simulink library "DatalogHandler"  (R2016b)
settings: Solver=VariableStepAuto  StartTime=0.0  StopTime=10.0  RelTol=1e-3
libraries: VariousLibrary x6, ConversionsLibrary x6, slrtlib x1
(part 1 of 2)
settings Model: Creator=march  LastModifiedBy=march

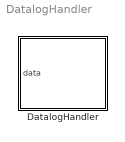
== system DatalogHandler ==
  DatalogHandler : Subsystem

== system DatalogHandler/DatalogHandler ==
  data : Inport
  Bus Selector1 : BusSelector  OutputSignals=etherCATData.receivedFromSOMANETs,etherCATData.sendToSOMANETs,miscDataSOMANETs.jointControlConfigs,miscDataSOMANETs.somanetData,etherCATData.receivedFromGESs,etherCATData.receivedFromInputDevice,etherCATData.sendToInputDevice,etherCATData.receivedFromPowerElectronics,etherCATData.sendToPowerElectronics,error,masterState,errorMessage
  "DataLogger " : slrtlib/Displays and Logging/Scope   scopeno=10  scopetype=File  autostart=on  viewmode=Graphical redraw  formatstr='%15.6f'  grid=on  ylimits=[0,0]  nosamples=900000  noprepostsamples=0  interleave=1  triggermode=FreeRun  triggersignal=1  trigsignalfromport=off  triggerlevel=0.0  triggerslope=Either  triggerscope=1  triggersample=0  filename=MARCH<%%>.dat  mode=Lazy  writesize=512  autorestart=on  dynamicfilemode=on  maxwritefilesize=512*1024^2
  Mux : Mux  Inputs=193
  Subsystem : Subsystem
  wires:
  Mux/1 -> "DataLogger "/1
  Subsystem/193(Out193) -> Mux/193
  Subsystem/192(Out192) -> Mux/192
  Subsystem/191(Out191) -> Mux/191
  Subsystem/190(Out190) -> Mux/190
  Subsystem/189(Out189) -> Mux/189
  Subsystem/188(Out188) -> Mux/188
  Subsystem/187(Out187) -> Mux/187
  Subsystem/186(Out186) -> Mux/186
  Subsystem/185(Out185) -> Mux/185
  Subsystem/184(Out184) -> Mux/184
  Subsystem/183(Out183) -> Mux/183
  Subsystem/182(Out182) -> Mux/182
  Subsystem/181(Out181) -> Mux/181
  Subsystem/180(Out180) -> Mux/180
  Subsystem/179(Out179) -> Mux/179
  Subsystem/178(Out178) -> Mux/178
  Subsystem/177(Out177) -> Mux/177
  Subsystem/176(Out176) -> Mux/176
  Subsystem/175(Out175) -> Mux/175
  Subsystem/174(Out174) -> Mux/174
  Subsystem/173(Out173) -> Mux/173
  Subsystem/172(Out172) -> Mux/172
  Subsystem/171(Out171) -> Mux/171
  Subsystem/170(Out170) -> Mux/170
  Subsystem/169(Out169) -> Mux/169
  Subsystem/168(Out168) -> Mux/168
  Subsystem/167(Out167) -> Mux/167
  Subsystem/166(Out166) -> Mux/166
  Subsystem/165(Out165) -> Mux/165
  Subsystem/164(Out164) -> Mux/164
  Subsystem/163(Out163) -> Mux/163
  Subsystem/162(Out162) -> Mux/162
  Subsystem/161(Out161) -> Mux/161
  Subsystem/160(Out160) -> Mux/160
  Subsystem/159(Out159) -> Mux/159
  Subsystem/158(Out158) -> Mux/158
  Subsystem/157(Out157) -> Mux/157
  Subsystem/156(Out156) -> Mux/156
  Subsystem/155(Out155) -> Mux/155
  Subsystem/154(Out154) -> Mux/154
  Subsystem/153(Out153) -> Mux/153
  Subsystem/152(Out152) -> Mux/152
  Subsystem/151(Out151) -> Mux/151
  Subsystem/150(Out150) -> Mux/150
  Subsystem/149(Out149) -> Mux/149
  Subsystem/148(Out148) -> Mux/148
  Subsystem/147(Out147) -> Mux/147
  Subsystem/146(Out146) -> Mux/146
  Subsystem/145(Out145) -> Mux/145
  Subsystem/144(Out144) -> Mux/144
  Subsystem/143(Out143) -> Mux/143
  Subsystem/142(Out142) -> Mux/142
  Subsystem/141(Out141) -> Mux/141
  Subsystem/140(Out140) -> Mux/140
  Subsystem/139(Out139) -> Mux/139
  Subsystem/138(Out138) -> Mux/138
  Subsystem/137(Out137) -> Mux/137
  Subsystem/136(Out136) -> Mux/136
  Subsystem/135(Out135) -> Mux/135
  Subsystem/134(Out134) -> Mux/134
  Subsystem/133(Out133) -> Mux/133
  Subsystem/132(Out132) -> Mux/132
  Subsystem/131(Out131) -> Mux/131
  Subsystem/130(Out130) -> Mux/130
  Subsystem/129(Out129) -> Mux/129
  Subsystem/128(Out128) -> Mux/128
  Subsystem/127(Out127) -> Mux/127
  Subsystem/126(Out126) -> Mux/126
  Subsystem/125(Out125) -> Mux/125
  Subsystem/124(Out124) -> Mux/124
  Subsystem/123(Out123) -> Mux/123
  Subsystem/122(Out122) -> Mux/122
  Subsystem/121(Out121) -> Mux/121
  Subsystem/120(Out120) -> Mux/120
  Subsystem/119(Out119) -> Mux/119
  Subsystem/118(Out118) -> Mux/118
  Subsystem/117(Out117) -> Mux/117
  Subsystem/116(Out116) -> Mux/116
  Subsystem/115(Out115) -> Mux/115
  Subsystem/114(Out114) -> Mux/114
  Subsystem/113(Out113) -> Mux/113
  Subsystem/112(Out112) -> Mux/112
  Subsystem/111(Out111) -> Mux/111
  Subsystem/110(Out110) -> Mux/110
  Subsystem/109(Out109) -> Mux/109
  Subsystem/108(Out108) -> Mux/108
  Subsystem/107(Out107) -> Mux/107
  Subsystem/106(Out106) -> Mux/106
  Subsystem/105(Out105) -> Mux/105
  Subsystem/104(Out104) -> Mux/104
  Subsystem/103(Out103) -> Mux/103
  Subsystem/102(Out102) -> Mux/102
  Subsystem/101(Out101) -> Mux/101
  Subsystem/100(Out100) -> Mux/100
  Subsystem/99(Out99) -> Mux/99
  Subsystem/98(Out98) -> Mux/98
  Subsystem/97(Out97) -> Mux/97
  Subsystem/96(Out96) -> Mux/96
  Subsystem/95(Out95) -> Mux/95
  Subsystem/94(Out94) -> Mux/94
  Subsystem/93(Out93) -> Mux/93
  Subsystem/92(Out92) -> Mux/92
  Subsystem/91(Out91) -> Mux/91
  Subsystem/90(Out90) -> Mux/90
  Subsystem/89(Out89) -> Mux/89
  Subsystem/88(Out88) -> Mux/88
  Subsystem/87(Out87) -> Mux/87
  Subsystem/86(Out86) -> Mux/86
  Subsystem/85(Out85) -> Mux/85
  Subsystem/84(Out84) -> Mux/84
  Subsystem/83(Out83) -> Mux/83
  Subsystem/82(Out82) -> Mux/82
  Subsystem/81(Out81) -> Mux/81
  Subsystem/80(Out80) -> Mux/80
  Subsystem/79(Out79) -> Mux/79
  Subsystem/78(Out78) -> Mux/78
  Subsystem/77(Out77) -> Mux/77
  Subsystem/76(Out76) -> Mux/76
  Subsystem/75(Out75) -> Mux/75
  Subsystem/74(Out74) -> Mux/74
  Subsystem/73(Out73) -> Mux/73
  Subsystem/72(Out72) -> Mux/72
  Subsystem/71(Out71) -> Mux/71
  Subsystem/70(Out70) -> Mux/70
  Subsystem/69(Out69) -> Mux/69
  Subsystem/68(Out68) -> Mux/68
  Subsystem/67(Out67) -> Mux/67
  Subsystem/66(Out66) -> Mux/66
  Subsystem/65(Out65) -> Mux/65
  Subsystem/64(Out64) -> Mux/64
  Subsystem/63(Out63) -> Mux/63
  Subsystem/62(Out62) -> Mux/62
  Subsystem/61(Out61) -> Mux/61
  Subsystem/60(Out60) -> Mux/60
  Subsystem/59(Out59) -> Mux/59
  Subsystem/58(Out58) -> Mux/58
  Subsystem/57(Out57) -> Mux/57
  Subsystem/56(Out56) -> Mux/56
  Subsystem/55(Out55) -> Mux/55
  Subsystem/54(Out54) -> Mux/54
  Subsystem/53(Out53) -> Mux/53
  Subsystem/52(Out52) -> Mux/52
  Subsystem/51(Out51) -> Mux/51
  Subsystem/50(Out50) -> Mux/50
  Subsystem/49(Out49) -> Mux/49
  Subsystem/48(Out48) -> Mux/48
  Subsystem/47(Out47) -> Mux/47
  Subsystem/46(Out46) -> Mux/46
  Subsystem/45(Out45) -> Mux/45
  Subsystem/44(Out44) -> Mux/44
  Subsystem/43(Out43) -> Mux/43
  Subsystem/42(Out42) -> Mux/42
  Subsystem/41(Out41) -> Mux/41
  Subsystem/40(Out40) -> Mux/40
  Subsystem/39(Out39) -> Mux/39
  Subsystem/38(Out38) -> Mux/38
  Subsystem/37(Out37) -> Mux/37
  Subsystem/36(Out36) -> Mux/36
  Subsystem/35(Out35) -> Mux/35
  Subsystem/34(Out34) -> Mux/34
  Subsystem/33(Out33) -> Mux/33
  Subsystem/32(Out32) -> Mux/32
  Subsystem/31(Out31) -> Mux/31
  Subsystem/30(Out30) -> Mux/30
  Subsystem/29(Out29) -> Mux/29
  Subsystem/28(Out28) -> Mux/28
  Subsystem/27(Out27) -> Mux/27
  Subsystem/26(Out26) -> Mux/26
  Subsystem/25(Out25) -> Mux/25
  Subsystem/24(Out24) -> Mux/24
  Subsystem/23(Out23) -> Mux/23
  Subsystem/22(Out22) -> Mux/22
  Subsystem/21(Out21) -> Mux/21
  Subsystem/20(Out20) -> Mux/20
  Subsystem/19(Out19) -> Mux/19
  Subsystem/18(Out18) -> Mux/18
  Subsystem/17(Out17) -> Mux/17
  Subsystem/16(Out16) -> Mux/16
  Subsystem/15(Out15) -> Mux/15
  Subsystem/14(Out14) -> Mux/14
  Subsystem/13(Out13) -> Mux/13
  Subsystem/12(Out12) -> Mux/12
  Subsystem/11(Out11) -> Mux/11
  Subsystem/10(Out10) -> Mux/10
  Subsystem/9(Out9) -> Mux/9
  Subsystem/8(Out8) -> Mux/8
  Subsystem/7(Out7) -> Mux/7
  Subsystem/6(Out6) -> Mux/6
  Subsystem/5(Out5) -> Mux/5
  Subsystem/4(Out4) -> Mux/4
  Subsystem/3(Out3) -> Mux/3
  Subsystem/2(Out2) -> Mux/2
  Subsystem/1(Out1) -> Mux/1
  Bus Selector1/12 -> Subsystem/12(In12)  "<errorMessage>"
  Bus Selector1/11 -> Subsystem/11(In11)  "<masterState>"
  Bus Selector1/10 -> Subsystem/10(In10)  "<error>"
  Bus Selector1/9 -> Subsystem/9(In9)  "<sendToPowerElectronics>"
  Bus Selector1/8 -> Subsystem/8(In8)  "<receivedFromPowerElectronics>"
  Bus Selector1/7 -> Subsystem/7(In7)  "<sendToInputDevice>"
  Bus Selector1/6 -> Subsystem/6(In6)  "<receivedFromInputDevice>"
  Bus Selector1/5 -> Subsystem/5(In5)  "<receivedFromGESs>"
  Bus Selector1/4 -> Subsystem/4(In4)  "<somanetData>"
  Bus Selector1/3 -> Subsystem/3(In3)  "<jointControlConfigs>"
  Bus Selector1/2 -> Subsystem/2(In2)  "<sendToSOMANETs>"
  Bus Selector1/1 -> Subsystem/1(In1)  "<receivedFromSOMANETs>"
  data/1 -> Bus Selector1/1

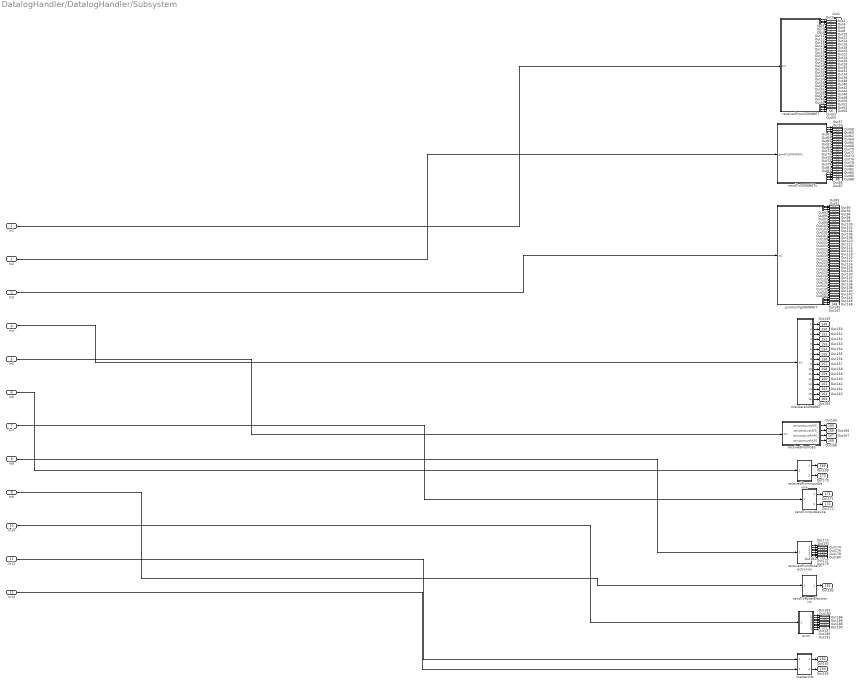
== system DatalogHandler/DatalogHandler/Subsystem ==
  In1 : Inport
  In2 : Inport  Port=2
  In3 : Inport  Port=3
  In4 : Inport  Port=4
  In5 : Inport  Port=5
  In6 : Inport  Port=6
  In7 : Inport  Port=7
  In8 : Inport  Port=8
  In9 : Inport  Port=9
  In10 : Inport  Port=10
  In11 : Inport  Port=11
  In12 : Inport  Port=12
  error : Subsystem
  jointConfigSOMANET : Subsystem
  masterInfo : Subsystem
  miscDataSOMANET : Subsystem
  receivedFromGES : Subsystem
  receivedFromInputDevice : Subsystem
  receivedFromPowerElectronics : Subsystem
  receivedFromSOMANET : Subsystem
  sendToInputDevice : Subsystem
  sendToPowerElectronics : Subsystem
  sendToSOMANETs : Subsystem
  Out1 : Outport
  Out2 : Outport  Port=2
  Out3 : Outport  Port=3
  Out4 : Outport  Port=4
  Out5 : Outport  Port=5
  Out6 : Outport  Port=6
  Out7 : Outport  Port=7
  Out8 : Outport  Port=8
  Out9 : Outport  Port=9
  Out10 : Outport  Port=10
  Out11 : Outport  Port=11
  Out12 : Outport  Port=12
  Out13 : Outport  Port=13
  Out14 : Outport  Port=14
  Out15 : Outport  Port=15
  Out16 : Outport  Port=16
  Out17 : Outport  Port=17
  Out18 : Outport  Port=18
  Out19 : Outport  Port=19
  Out20 : Outport  Port=20
  Out21 : Outport  Port=21
  Out22 : Outport  Port=22
  Out23 : Outport  Port=23
  Out24 : Outport  Port=24
  Out25 : Outport  Port=25
  Out26 : Outport  Port=26
  Out27 : Outport  Port=27
  Out28 : Outport  Port=28
  Out29 : Outport  Port=29
  Out30 : Outport  Port=30
  Out31 : Outport  Port=31
  Out32 : Outport  Port=32
  Out33 : Outport  Port=33
  Out34 : Outport  Port=34
  Out35 : Outport  Port=35
  Out36 : Outport  Port=36
  Out37 : Outport  Port=37
  Out38 : Outport  Port=38
  Out39 : Outport  Port=39
  Out40 : Outport  Port=40
  Out41 : Outport  Port=41
  Out42 : Outport  Port=42
  Out43 : Outport  Port=43
  Out44 : Outport  Port=44
  Out45 : Outport  Port=45
  Out46 : Outport  Port=46
  Out47 : Outport  Port=47
  Out48 : Outport  Port=48
  Out49 : Outport  Port=49
  Out50 : Outport  Port=50
  Out51 : Outport  Port=51
  Out52 : Outport  Port=52
  Out53 : Outport  Port=53
  Out54 : Outport  Port=54
  Out55 : Outport  Port=55
  Out56 : Outport  Port=56
  Out57 : Outport  Port=57
  Out58 : Outport  Port=58
  Out59 : Outport  Port=59
  Out60 : Outport  Port=60
  Out61 : Outport  Port=61
  Out62 : Outport  Port=62
  Out63 : Outport  Port=63
  Out64 : Outport  Port=64
  Out65 : Outport  Port=65
  Out66 : Outport  Port=66
  Out67 : Outport  Port=67
  Out68 : Outport  Port=68
  Out69 : Outport  Port=69
  Out70 : Outport  Port=70
  Out71 : Outport  Port=71
  Out72 : Outport  Port=72
  Out73 : Outport  Port=73
  Out74 : Outport  Port=74
  Out75 : Outport  Port=75
  Out76 : Outport  Port=76
  Out77 : Outport  Port=77
  Out78 : Outport  Port=78
  Out79 : Outport  Port=79
  Out80 : Outport  Port=80
  Out81 : Outport  Port=81
  Out82 : Outport  Port=82
  Out83 : Outport  Port=83
  Out84 : Outport  Port=84
  Out85 : Outport  Port=85
  Out86 : Outport  Port=86
  Out87 : Outport  Port=87
  Out88 : Outport  Port=88
  Out89 : Outport  Port=89
  Out90 : Outport  Port=90
  Out91 : Outport  Port=91
  Out92 : Outport  Port=92
  Out93 : Outport  Port=93
  Out94 : Outport  Port=94
  Out95 : Outport  Port=95
  Out96 : Outport  Port=96
  Out97 : Outport  Port=97
  Out98 : Outport  Port=98
  Out99 : Outport  Port=99
  Out100 : Outport  Port=100
  Out101 : Outport  Port=101
  Out102 : Outport  Port=102
  Out103 : Outport  Port=103
  Out104 : Outport  Port=104
  Out105 : Outport  Port=105
  Out106 : Outport  Port=106
  Out107 : Outport  Port=107
  Out108 : Outport  Port=108
  Out109 : Outport  Port=109
  Out110 : Outport  Port=110
  Out111 : Outport  Port=111
  Out112 : Outport  Port=112
  Out113 : Outport  Port=113
  Out114 : Outport  Port=114
  Out115 : Outport  Port=115
  Out116 : Outport  Port=116
  Out117 : Outport  Port=117
  Out118 : Outport  Port=118
  Out119 : Outport  Port=119
  Out120 : Outport  Port=120
  Out121 : Outport  Port=121
  Out122 : Outport  Port=122
  Out123 : Outport  Port=123
  Out124 : Outport  Port=124
  Out125 : Outport  Port=125
  Out126 : Outport  Port=126
  Out127 : Outport  Port=127
  Out128 : Outport  Port=128
  Out129 : Outport  Port=129
  Out130 : Outport  Port=130
  Out131 : Outport  Port=131
  Out132 : Outport  Port=132
  Out133 : Outport  Port=133
  Out134 : Outport  Port=134
  Out135 : Outport  Port=135
  Out136 : Outport  Port=136
  Out137 : Outport  Port=137
  Out138 : Outport  Port=138
  Out139 : Outport  Port=139
  Out140 : Outport  Port=140
  Out141 : Outport  Port=141
  Out142 : Outport  Port=142
  Out143 : Outport  Port=143
  Out144 : Outport  Port=144
  Out145 : Outport  Port=145
  Out146 : Outport  Port=146
  Out147 : Outport  Port=147
  Out148 : Outport  Port=148
  Out149 : Outport  Port=149
  Out150 : Outport  Port=150
  Out151 : Outport  Port=151
  Out152 : Outport  Port=152
  Out153 : Outport  Port=153
  Out154 : Outport  Port=154
  Out155 : Outport  Port=155
  Out156 : Outport  Port=156
  Out157 : Outport  Port=157
  Out158 : Outport  Port=158
  Out159 : Outport  Port=159
  Out160 : Outport  Port=160
  Out161 : Outport  Port=161
  Out162 : Outport  Port=162
  Out163 : Outport  Port=163
  Out164 : Outport  Port=164
  Out165 : Outport  Port=165
  Out166 : Outport  Port=166
  Out167 : Outport  Port=167
  Out168 : Outport  Port=168
  Out169 : Outport  Port=169
  Out170 : Outport  Port=170
  Out171 : Outport  Port=171
  Out172 : Outport  Port=172
  Out173 : Outport  Port=173
  Out174 : Outport  Port=174
  Out175 : Outport  Port=175
  Out176 : Outport  Port=176
  Out177 : Outport  Port=177
  Out178 : Outport  Port=178
  Out179 : Outport  Port=179
  Out180 : Outport  Port=180
  Out181 : Outport  Port=181
  Out182 : Outport  Port=182
  Out183 : Outport  Port=183
  Out184 : Outport  Port=184
  Out185 : Outport  Port=185
  Out186 : Outport  Port=186
  Out187 : Outport  Port=187
  Out188 : Outport  Port=188
  Out189 : Outport  Port=189
  Out190 : Outport  Port=190
  Out191 : Outport  Port=191
  Out192 : Outport  Port=192
  Out193 : Outport  Port=193
  wires:
  In12/1 -> masterInfo/2(In2)
  In2/1 -> sendToSOMANETs/1(sendToSOMANETs)
  In6/1 -> receivedFromInputDevice/1(In1)
  In3/1 -> jointConfigSOMANET/1(In1)
  In11/1 -> masterInfo/1(In1)
  In10/1 -> error/1(In1)
  In9/1 -> sendToPowerElectronics/1(In1)
  In7/1 -> sendToInputDevice/1(In1)
  In8/1 -> receivedFromPowerElectronics/1(In1)
  In1/1 -> receivedFromSOMANET/1(In1)
  In5/1 -> receivedFromGES/1(In1)
  In4/1 -> miscDataSOMANET/1(In1)
  error/1(Out1) -> Out183/1
  masterInfo/2(Out2) -> Out193/1
  miscDataSOMANET/14(Out11) -> Out162/1
  masterInfo/1(Out1) -> Out192/1
  miscDataSOMANET/8(Out14) -> Out156/1
  miscDataSOMANET/16(Out16) -> Out164/1
  miscDataSOMANET/11(Out9) -> Out159/1
  error/7(Out4) -> Out189/1
  error/6(Out3) -> Out188/1
  miscDataSOMANET/10(Out8) -> Out158/1
  miscDataSOMANET/6(Out5) -> Out154/1
  miscDataSOMANET/9(Out7) -> Out157/1
  miscDataSOMANET/12(Out15) -> Out160/1
  miscDataSOMANET/15(Out12) -> Out163/1
  miscDataSOMANET/7(Out6) -> Out155/1
  error/9(Out8) -> Out191/1
  miscDataSOMANET/13(Out10) -> Out161/1
  error/8(Out9) -> Out190/1
  miscDataSOMANET/2(Out2) -> Out150/1
  receivedFromSOMANET/42(Out42) -> Out42/1
  miscDataSOMANET/5(Out4) -> Out153/1
  receivedFromSOMANET/47(Out47) -> Out47/1
  receivedFromSOMANET/39(Out39) -> Out39/1
  receivedFromSOMANET/44(Out44) -> Out44/1
  miscDataSOMANET/4(Out13) -> Out152/1
  receivedFromSOMANET/35(Out35) -> Out35/1
  receivedFromSOMANET/43(Out43) -> Out43/1
  receivedFromSOMANET/41(Out41) -> Out41/1
  receivedFromSOMANET/46(Out46) -> Out46/1
  receivedFromGES/4(temperatureRKFE_) -> Out168/1
  receivedFromGES/3(temperatureRHFE_) -> Out167/1
  receivedFromSOMANET/48(Out48) -> Out48/1
  receivedFromSOMANET/45(Out45) -> Out45/1
  receivedFromSOMANET/40(Out40) -> Out40/1
  receivedFromSOMANET/38(Out38) -> Out38/1
  miscDataSOMANET/3(Out3) -> Out151/1
  miscDataSOMANET/1(Out1) -> Out149/1
  receivedFromSOMANET/37(Out37) -> Out37/1
  receivedFromSOMANET/36(Out36) -> Out36/1
  jointConfigSOMANET/57(Out57) -> Out145/1
  receivedFromSOMANET/21(Out21) -> Out21/1
  sendToSOMANETs/3(Out3) -> Out59/1
  receivedFromSOMANET/32(Out32) -> Out32/1
  receivedFromSOMANET/30(Out30) -> Out30/1
  receivedFromSOMANET/28(Out28) -> Out28/1
  receivedFromSOMANET/29(Out29) -> Out29/1
  receivedFromSOMANET/23(Out23) -> Out23/1
  receivedFromSOMANET/18(Out18) -> Out18/1
  sendToSOMANETs/4(Out4) -> Out60/1
  receivedFromSOMANET/27(Out27) -> Out27/1
  jointConfigSOMANET/60(Out60) -> Out148/1
  jointConfigSOMANET/58(Out58) -> Out146/1
  receivedFromSOMANET/25(Out25) -> Out25/1
  receivedFromSOMANET/22(Out22) -> Out22/1
  receivedFromGES/2(temperatureLKFE_) -> Out166/1
  sendToSOMANETs/5(Out5) -> Out61/1
  jointConfigSOMANET/59(Out59) -> Out147/1
  receivedFromSOMANET/19(Out19) -> Out19/1
  sendToSOMANETs/1(Out1) -> Out57/1
  receivedFromSOMANET/34(Out34) -> Out34/1
  receivedFromSOMANET/31(Out31) -> Out31/1
  receivedFromSOMANET/33(Out33) -> Out33/1
  receivedFromSOMANET/26(Out26) -> Out26/1
  receivedFromSOMANET/20(Out20) -> Out20/1
  jointConfigSOMANET/54(Out54) -> Out142/1
  jointConfigSOMANET/55(Out55) -> Out143/1
  jointConfigSOMANET/56(Out56) -> Out144/1
  jointConfigSOMANET/16(Out16) -> Out104/1
  jointConfigSOMANET/15(Out15) -> Out103/1
  jointConfigSOMANET/14(Out14) -> Out102/1
  jointConfigSOMANET/13(Out13) -> Out101/1
  jointConfigSOMANET/5(Out5) -> Out93/1
  jointConfigSOMANET/6(Out6) -> Out94/1
  jointConfigSOMANET/12(Out12) -> Out100/1
  jointConfigSOMANET/11(Out11) -> Out99/1
  jointConfigSOMANET/8(Out8) -> Out96/1
  jointConfigSOMANET/10(Out10) -> Out98/1
  jointConfigSOMANET/9(Out9) -> Out97/1
  jointConfigSOMANET/7(Out7) -> Out95/1
  receivedFromSOMANET/1(Out1) -> Out1/1
  receivedFromSOMANET/9(Out9) -> Out9/1
  receivedFromSOMANET/10(Out10) -> Out10/1
  receivedFromSOMANET/11(Out11) -> Out11/1
  error/5(Out2) -> Out187/1
  receivedFromSOMANET/12(Out12) -> Out12/1
  error/2(Out5) -> Out184/1
  error/4(Out7) -> Out186/1
  receivedFromSOMANET/13(Out13) -> Out13/1
  receivedFromSOMANET/8(Out8) -> Out8/1
  error/3(Out6) -> Out185/1
  receivedFromSOMANET/15(Out15) -> Out15/1
  receivedFromSOMANET/17(Out17) -> Out17/1
  receivedFromSOMANET/16(Out16) -> Out16/1
  receivedFromSOMANET/14(Out14) -> Out14/1
  sendToSOMANETs/10(Out10) -> Out66/1
  sendToSOMANETs/11(Out11) -> Out67/1
  sendToSOMANETs/23(Out23) -> Out79/1
  receivedFromSOMANET/7(Out7) -> Out7/1
  receivedFromSOMANET/6(Out6) -> Out6/1
  sendToSOMANETs/21(Out21) -> Out77/1
  sendToSOMANETs/18(Out18) -> Out74/1
  sendToSOMANETs/17(Out17) -> Out73/1
  receivedFromSOMANET/5(Out5) -> Out5/1
  sendToSOMANETs/24(Out24) -> Out80/1
  sendToSOMANETs/20(Out20) -> Out76/1
  sendToSOMANETs/32(Out32) -> Out88/1
  receivedFromSOMANET/4(Out4) -> Out4/1
  receivedFromSOMANET/3(Out3) -> Out3/1
  receivedFromSOMANET/2(Out2) -> Out2/1
  sendToSOMANETs/30(Out30) -> Out86/1
  sendToSOMANETs/26(Out26) -> Out82/1
  sendToSOMANETs/28(Out28) -> Out84/1
  sendToSOMANETs/19(Out19) -> Out75/1
  sendToSOMANETs/13(Out13) -> Out69/1
  sendToSOMANETs/22(Out22) -> Out78/1
  sendToSOMANETs/29(Out29) -> Out85/1
  sendToSOMANETs/14(Out14) -> Out70/1
  sendToSOMANETs/16(Out16) -> Out72/1
  sendToSOMANETs/12(Out12) -> Out68/1
  sendToPowerElectronics/1(Out1) -> Out182/1
  sendToSOMANETs/25(Out25) -> Out81/1
  sendToSOMANETs/31(Out31) -> Out87/1
  sendToSOMANETs/15(Out15) -> Out71/1
  sendToSOMANETs/27(Out27) -> Out83/1
  jointConfigSOMANET/32(Out32) -> Out120/1
  jointConfigSOMANET/47(Out47) -> Out135/1
  jointConfigSOMANET/39(Out39) -> Out127/1
  jointConfigSOMANET/34(Out34) -> Out122/1
  jointConfigSOMANET/35(Out35) -> Out123/1
  jointConfigSOMANET/30(Out30) -> Out118/1
  jointConfigSOMANET/52(Out52) -> Out140/1
  jointConfigSOMANET/50(Out50) -> Out138/1
  jointConfigSOMANET/36(Out36) -> Out124/1
  jointConfigSOMANET/40(Out40) -> Out128/1
  jointConfigSOMANET/42(Out42) -> Out130/1
  sendToSOMANETs/9(Out9) -> Out65/1
  jointConfigSOMANET/41(Out41) -> Out129/1
  jointConfigSOMANET/45(Out45) -> Out133/1
  jointConfigSOMANET/44(Out44) -> Out132/1
  jointConfigSOMANET/38(Out38) -> Out126/1
  jointConfigSOMANET/33(Out33) -> Out121/1
  jointConfigSOMANET/31(Out31) -> Out119/1
  jointConfigSOMANET/43(Out43) -> Out131/1
  jointConfigSOMANET/53(Out53) -> Out141/1
  jointConfigSOMANET/51(Out51) -> Out139/1
  jointConfigSOMANET/37(Out37) -> Out125/1
  jointConfigSOMANET/49(Out49) -> Out137/1
  jointConfigSOMANET/46(Out46) -> Out134/1
  jointConfigSOMANET/29(Out29) -> Out117/1
  jointConfigSOMANET/48(Out48) -> Out136/1
  jointConfigSOMANET/25(Out25) -> Out113/1
  jointConfigSOMANET/18(Out18) -> Out106/1
  jointConfigSOMANET/21(Out21) -> Out109/1
  jointConfigSOMANET/17(Out17) -> Out105/1
  jointConfigSOMANET/19(Out19) -> Out107/1
  jointConfigSOMANET/26(Out26) -> Out114/1
  jointConfigSOMANET/24(Out24) -> Out112/1
  jointConfigSOMANET/22(Out22) -> Out110/1
  jointConfigSOMANET/20(Out20) -> Out108/1
  jointConfigSOMANET/23(Out23) -> Out111/1
  jointConfigSOMANET/28(Out28) -> Out116/1
  jointConfigSOMANET/27(Out27) -> Out115/1
  receivedFromSOMANET/51(Out51) -> Out51/1
  receivedFromSOMANET/56(Out56) -> Out56/1
  receivedFromSOMANET/53(Out53) -> Out53/1
  receivedFromGES/1(temperatureLHFE_) -> Out165/1
  receivedFromPowerElectronics/6(Out6) -> Out178/1
  receivedFromSOMANET/54(Out54) -> Out54/1
  receivedFromInputDevice/2(Out2) -> Out170/1
  receivedFromInputDevice/1(Out1) -> Out169/1
  receivedFromPowerElectronics/4(Out4) -> Out176/1
  receivedFromPowerElectronics/1(Out1) -> Out173/1
  receivedFromSOMANET/55(Out55) -> Out55/1
  receivedFromPowerElectronics/7(Out7) -> Out179/1
  receivedFromPowerElectronics/9(Out9) -> Out181/1
  receivedFromPowerElectronics/8(Out8) -> Out180/1
  receivedFromPowerElectronics/5(Out5) -> Out177/1
  receivedFromSOMANET/52(Out52) -> Out52/1
  receivedFromPowerElectronics/3(Out3) -> Out175/1
  receivedFromPowerElectronics/2(Out2) -> Out174/1
  jointConfigSOMANET/2(Out2) -> Out90/1
  receivedFromSOMANET/24(Out24) -> Out24/1
  sendToSOMANETs/6(Out6) -> Out62/1
  sendToSOMANETs/8(Out8) -> Out64/1
  sendToSOMANETs/7(Out7) -> Out63/1
  sendToSOMANETs/2(Out2) -> Out58/1
  jointConfigSOMANET/1(Out1) -> Out89/1
  sendToInputDevice/2(Out2) -> Out172/1
  jointConfigSOMANET/4(Out4) -> Out92/1
  jointConfigSOMANET/3(Out3) -> Out91/1
  sendToInputDevice/1(Out1) -> Out171/1
  receivedFromSOMANET/50(Out50) -> Out50/1
  receivedFromSOMANET/49(Out49) -> Out49/1

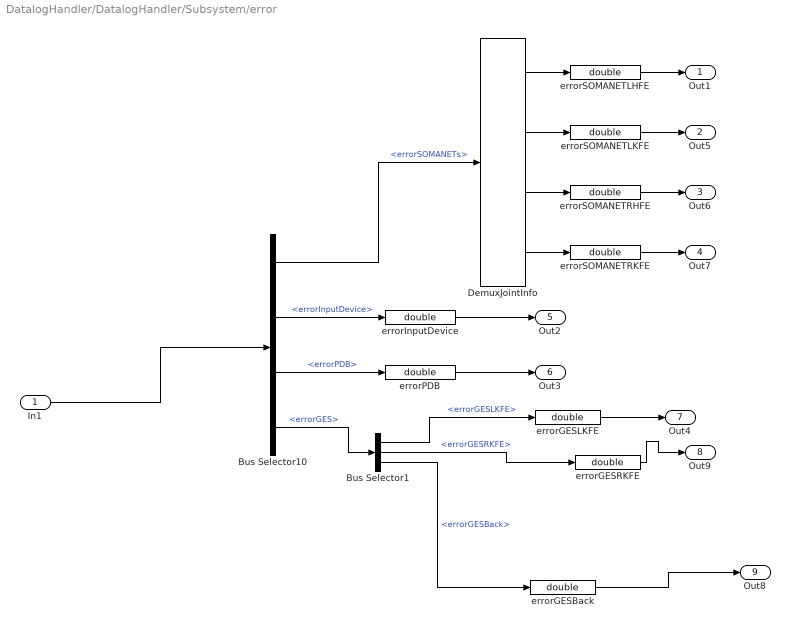
== system DatalogHandler/DatalogHandler/Subsystem/error ==
  In1 : Inport
  Bus Selector1 : BusSelector  OutputSignals=errorGESLKFE,errorGESRKFE,errorGESBack
  Bus Selector10 : BusSelector  OutputSignals=errorSOMANETs,errorInputDevice,errorPowerElectronics.errorPDB,errorGES
  DemuxJointInfo : VariousLibrary/DemuxJointInfo
  errorGESBack : DataTypeConversion  OutDataTypeStr=double  RndMeth=Nearest
  errorGESLKFE : DataTypeConversion  OutDataTypeStr=double  RndMeth=Nearest
  errorGESRKFE : DataTypeConversion  OutDataTypeStr=double  RndMeth=Nearest
  errorInputDevice : DataTypeConversion  OutDataTypeStr=double  RndMeth=Nearest
  errorPDB : DataTypeConversion  OutDataTypeStr=double  RndMeth=Nearest
  errorSOMANETLHFE : DataTypeConversion  OutDataTypeStr=double  RndMeth=Nearest
  errorSOMANETLKFE : DataTypeConversion  OutDataTypeStr=double  RndMeth=Nearest
  errorSOMANETRHFE : DataTypeConversion  OutDataTypeStr=double  RndMeth=Nearest
  errorSOMANETRKFE : DataTypeConversion  OutDataTypeStr=double  RndMeth=Nearest
  Out1 : Outport
  Out5 : Outport  Port=2
  Out6 : Outport  Port=3
  Out7 : Outport  Port=4
  Out2 : Outport  Port=5
  Out3 : Outport  Port=6
  Out4 : Outport  Port=7
  Out9 : Outport  Port=8
  Out8 : Outport  Port=9
  wires:
  errorGESBack/1 -> Out8/1
  errorGESRKFE/1 -> Out9/1
  errorGESLKFE/1 -> Out4/1
  Bus Selector1/2 -> errorGESRKFE/1  "<errorGESRKFE>"
  Bus Selector1/3 -> errorGESBack/1  "<errorGESBack>"
  Bus Selector1/1 -> errorGESLKFE/1  "<errorGESLKFE>"
  Bus Selector10/4 -> Bus Selector1/1  "<errorGES>"
  errorSOMANETRKFE/1 -> Out7/1
  errorSOMANETRHFE/1 -> Out6/1
  errorSOMANETLKFE/1 -> Out5/1
  errorSOMANETLHFE/1 -> Out1/1
  DemuxJointInfo/2 -> errorSOMANETLKFE/1
  DemuxJointInfo/3 -> errorSOMANETRHFE/1
  DemuxJointInfo/4 -> errorSOMANETRKFE/1
  errorPDB/1 -> Out3/1
  errorInputDevice/1 -> Out2/1
  DemuxJointInfo/1 -> errorSOMANETLHFE/1
  In1/1 -> Bus Selector10/1
  Bus Selector10/3 -> errorPDB/1  "<errorPDB>"
  Bus Selector10/1 -> DemuxJointInfo/1  "<errorSOMANETs>"
  Bus Selector10/2 -> errorInputDevice/1  "<errorInputDevice>"

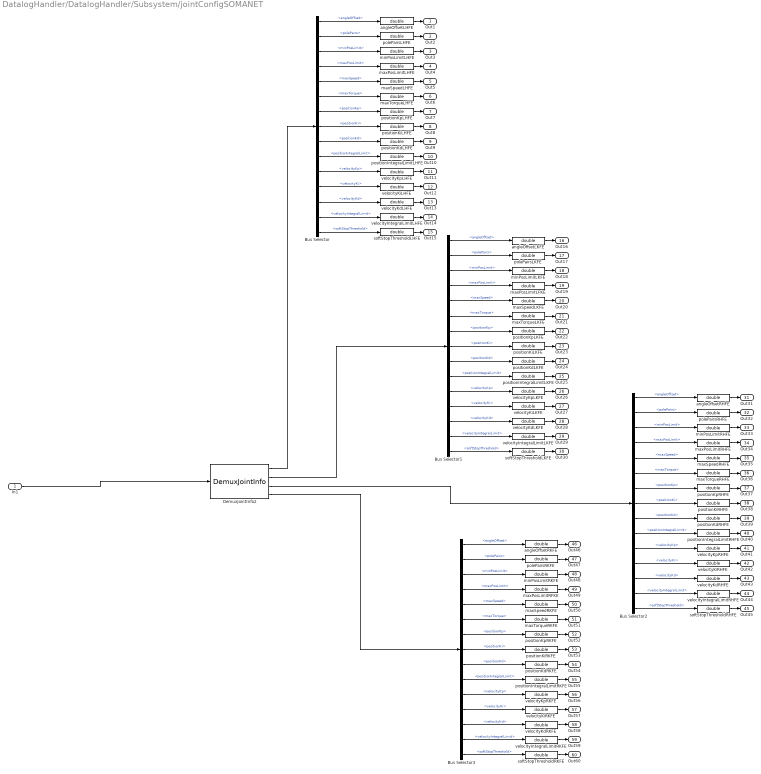
== system DatalogHandler/DatalogHandler/Subsystem/jointConfigSOMANET ==
  In1 : Inport
  Bus Selector{,1..3} (4 alike) : BusSelector  OutputSignals=angleOffset,polePairs,minPosLimit,maxPosLimit,maxSpeed,maxTorque,positionKp,positionKi,positionKd,positionIntegralLimit,velocityKp,velocityKi,velocityKd,velocityIntegralLimit,softStopThreshold
  DemuxJointInfo2 : VariousLibrary/DemuxJointInfo
  angleOffsetLHFE : DataTypeConversion  OutDataTypeStr=double  RndMeth=Nearest
  angleOffsetLKFE : DataTypeConversion  OutDataTypeStr=double  RndMeth=Nearest
  angleOffsetRHFE : DataTypeConversion  OutDataTypeStr=double  RndMeth=Nearest
  angleOffsetRKFE : DataTypeConversion  OutDataTypeStr=double  RndMeth=Nearest
  maxPosLimitLFKE : DataTypeConversion  OutDataTypeStr=double  RndMeth=Nearest
  maxPosLimitLHFE : DataTypeConversion  OutDataTypeStr=double  RndMeth=Nearest
  maxPosLimitRFKE : DataTypeConversion  OutDataTypeStr=double  RndMeth=Nearest
  maxPosLimitRHFE : DataTypeConversion  OutDataTypeStr=double  RndMeth=Nearest
  maxSpeedLHFE : DataTypeConversion  OutDataTypeStr=double  RndMeth=Nearest
  maxSpeedLKFE : DataTypeConversion  OutDataTypeStr=double  RndMeth=Nearest
  maxSpeedRHFE : DataTypeConversion  OutDataTypeStr=double  RndMeth=Nearest
  maxSpeedRKFE : DataTypeConversion  OutDataTypeStr=double  RndMeth=Nearest
  maxTorqueLHFE : DataTypeConversion  OutDataTypeStr=double  RndMeth=Nearest
  maxTorqueLKFE : DataTypeConversion  OutDataTypeStr=double  RndMeth=Nearest
  maxTorqueRHFE : DataTypeConversion  OutDataTypeStr=double  RndMeth=Nearest
  maxTorqueRKFE : DataTypeConversion  OutDataTypeStr=double  RndMeth=Nearest
  minPosLimitLHFE : DataTypeConversion  OutDataTypeStr=double  RndMeth=Nearest
  minPosLimitLKFE : DataTypeConversion  OutDataTypeStr=double  RndMeth=Nearest
  minPosLimitRHFE : DataTypeConversion  OutDataTypeStr=double  RndMeth=Nearest
  minPosLimitRKFE : DataTypeConversion  OutDataTypeStr=double  RndMeth=Nearest
  polePairsLHFE : DataTypeConversion  OutDataTypeStr=double  RndMeth=Nearest
  polePairsLKFE : DataTypeConversion  OutDataTypeStr=double  RndMeth=Nearest
  polePairsRHFE : DataTypeConversion  OutDataTypeStr=double  RndMeth=Nearest
  polePairsRKFE : DataTypeConversion  OutDataTypeStr=double  RndMeth=Nearest
  positionIntegralLimitLHFE : DataTypeConversion  OutDataTypeStr=double  RndMeth=Nearest
  positionIntegralLimitLKFE : DataTypeConversion  OutDataTypeStr=double  RndMeth=Nearest
  positionIntegralLimitRHFE : DataTypeConversion  OutDataTypeStr=double  RndMeth=Nearest
  positionIntegralLimitRKFE : DataTypeConversion  OutDataTypeStr=double  RndMeth=Nearest
  positionKdLHFE : DataTypeConversion  OutDataTypeStr=double  RndMeth=Nearest
  positionKdLKFE : DataTypeConversion  OutDataTypeStr=double  RndMeth=Nearest
  positionKdRHFE : DataTypeConversion  OutDataTypeStr=double  RndMeth=Nearest
  positionKdRKFE : DataTypeConversion  OutDataTypeStr=double  RndMeth=Nearest
  positionKiLHFE : DataTypeConversion  OutDataTypeStr=double  RndMeth=Nearest
  positionKiLKFE : DataTypeConversion  OutDataTypeStr=double  RndMeth=Nearest
  "positionKiRHFE " : DataTypeConversion  OutDataTypeStr=double  RndMeth=Nearest
  positionKiRKFE : DataTypeConversion  OutDataTypeStr=double  RndMeth=Nearest
  positionKpLHFE : DataTypeConversion  OutDataTypeStr=double  RndMeth=Nearest
  positionKpLKFE : DataTypeConversion  OutDataTypeStr=double  RndMeth=Nearest
  positionKpRHFE : DataTypeConversion  OutDataTypeStr=double  RndMeth=Nearest
  positionKpRKFE : DataTypeConversion  OutDataTypeStr=double  RndMeth=Nearest
  softStopThresholdLHFE : DataTypeConversion  OutDataTypeStr=double  RndMeth=Nearest
  softStopThresholdLKFE : DataTypeConversion  OutDataTypeStr=double  RndMeth=Nearest
  softStopThresholdRHFE : DataTypeConversion  OutDataTypeStr=double  RndMeth=Nearest
  softStopThresholdRKFE : DataTypeConversion  OutDataTypeStr=double  RndMeth=Nearest
  velocityIntegralLimitLHFE : DataTypeConversion  OutDataTypeStr=double  RndMeth=Nearest
  velocityIntegralLimitLKFE : DataTypeConversion  OutDataTypeStr=double  RndMeth=Nearest
  velocityIntegralLimitRHFE : DataTypeConversion  OutDataTypeStr=double  RndMeth=Nearest
  velocityIntegralLimitRKFE : DataTypeConversion  OutDataTypeStr=double  RndMeth=Nearest
  velocityKdLHFE : DataTypeConversion  OutDataTypeStr=double  RndMeth=Nearest
  velocityKdLKFE : DataTypeConversion  OutDataTypeStr=double  RndMeth=Nearest
  velocityKdRHFE : DataTypeConversion  OutDataTypeStr=double  RndMeth=Nearest
  velocityKdRKFE : DataTypeConversion  OutDataTypeStr=double  RndMeth=Nearest
  velocityKiLHFE : DataTypeConversion  OutDataTypeStr=double  RndMeth=Nearest
  velocityKiLKFE : DataTypeConversion  OutDataTypeStr=double  RndMeth=Nearest
  velocityKiRHFE : DataTypeConversion  OutDataTypeStr=double  RndMeth=Nearest
  velocityKiRKFE : DataTypeConversion  OutDataTypeStr=double  RndMeth=Nearest
  velocityKpLHFE : DataTypeConversion  OutDataTypeStr=double  RndMeth=Nearest
  velocityKpLKFE : DataTypeConversion  OutDataTypeStr=double  RndMeth=Nearest
  velocityKpRHFE : DataTypeConversion  OutDataTypeStr=double  RndMeth=Nearest
  velocityKpRKFE : DataTypeConversion  OutDataTypeStr=double  RndMeth=Nearest
  Out1 : Outport
  Out2 : Outport  Port=2
  Out3 : Outport  Port=3
  Out4 : Outport  Port=4
  Out5 : Outport  Port=5
  Out6 : Outport  Port=6
  Out7 : Outport  Port=7
  Out8 : Outport  Port=8
  Out9 : Outport  Port=9
  Out10 : Outport  Port=10
  Out11 : Outport  Port=11
  Out12 : Outport  Port=12
  Out13 : Outport  Port=13
  Out14 : Outport  Port=14
  Out15 : Outport  Port=15
  Out16 : Outport  Port=16
  Out17 : Outport  Port=17
  Out18 : Outport  Port=18
  Out19 : Outport  Port=19
  Out20 : Outport  Port=20
  Out21 : Outport  Port=21
  Out22 : Outport  Port=22
  Out23 : Outport  Port=23
  Out24 : Outport  Port=24
  Out25 : Outport  Port=25
  Out26 : Outport  Port=26
  Out27 : Outport  Port=27
  Out28 : Outport  Port=28
  Out29 : Outport  Port=29
  Out30 : Outport  Port=30
  Out31 : Outport  Port=31
  Out32 : Outport  Port=32
  Out33 : Outport  Port=33
  Out34 : Outport  Port=34
  Out35 : Outport  Port=35
  Out36 : Outport  Port=36
  Out37 : Outport  Port=37
  Out38 : Outport  Port=38
  Out39 : Outport  Port=39
  Out40 : Outport  Port=40
  Out41 : Outport  Port=41
  Out42 : Outport  Port=42
  Out43 : Outport  Port=43
  Out44 : Outport  Port=44
  Out45 : Outport  Port=45
  Out46 : Outport  Port=46
  Out47 : Outport  Port=47
  Out48 : Outport  Port=48
  Out49 : Outport  Port=49
  Out50 : Outport  Port=50
  Out51 : Outport  Port=51
  Out52 : Outport  Port=52
  Out53 : Outport  Port=53
  Out54 : Outport  Port=54
  Out55 : Outport  Port=55
  Out56 : Outport  Port=56
  Out57 : Outport  Port=57
  Out58 : Outport  Port=58
  Out59 : Outport  Port=59
  Out60 : Outport  Port=60
  wires:
  softStopThresholdRKFE/1 -> Out60/1
  velocityIntegralLimitRKFE/1 -> Out59/1
  velocityKdRKFE/1 -> Out58/1
  velocityKiRKFE/1 -> Out57/1
  velocityKpRKFE/1 -> Out56/1
  positionIntegralLimitRKFE/1 -> Out55/1
  positionKdRKFE/1 -> Out54/1
  positionKiRKFE/1 -> Out53/1
  positionKpRKFE/1 -> Out52/1
  maxTorqueRKFE/1 -> Out51/1
  maxSpeedRKFE/1 -> Out50/1
  maxPosLimitRFKE/1 -> Out49/1
  minPosLimitRKFE/1 -> Out48/1
  polePairsRKFE/1 -> Out47/1
  angleOffsetRKFE/1 -> Out46/1
  Bus Selector3/15 -> softStopThresholdRKFE/1  "<softStopThreshold>"
  Bus Selector3/14 -> velocityIntegralLimitRKFE/1  "<velocityIntegralLimit>"
  Bus Selector3/13 -> velocityKdRKFE/1  "<velocityKd>"
  Bus Selector3/12 -> velocityKiRKFE/1  "<velocityKi>"
  Bus Selector3/11 -> velocityKpRKFE/1  "<velocityKp>"
  Bus Selector3/10 -> positionIntegralLimitRKFE/1  "<positionIntegralLimit>"
  Bus Selector3/9 -> positionKdRKFE/1  "<positionKd>"
  Bus Selector3/8 -> positionKiRKFE/1  "<positionKi>"
  Bus Selector3/7 -> positionKpRKFE/1  "<positionKp>"
  Bus Selector3/6 -> maxTorqueRKFE/1  "<maxTorque>"
  Bus Selector3/5 -> maxSpeedRKFE/1  "<maxSpeed>"
  Bus Selector3/4 -> maxPosLimitRFKE/1  "<maxPosLimit>"
  Bus Selector3/3 -> minPosLimitRKFE/1  "<minPosLimit>"
  Bus Selector3/2 -> polePairsRKFE/1  "<polePairs>"
  Bus Selector3/1 -> angleOffsetRKFE/1  "<angleOffset>"
  DemuxJointInfo2/4 -> Bus Selector3/1
  softStopThresholdRHFE/1 -> Out45/1
  velocityIntegralLimitRHFE/1 -> Out44/1
  velocityKdRHFE/1 -> Out43/1
  velocityKiRHFE/1 -> Out42/1
  velocityKpRHFE/1 -> Out41/1
  positionIntegralLimitRHFE/1 -> Out40/1
  positionKdRHFE/1 -> Out39/1
  "positionKiRHFE "/1 -> Out38/1
  positionKpRHFE/1 -> Out37/1
  maxTorqueRHFE/1 -> Out36/1
  maxSpeedRHFE/1 -> Out35/1
  maxPosLimitRHFE/1 -> Out34/1
  minPosLimitRHFE/1 -> Out33/1
  polePairsRHFE/1 -> Out32/1
  angleOffsetRHFE/1 -> Out31/1
  Bus Selector2/15 -> softStopThresholdRHFE/1  "<softStopThreshold>"
  Bus Selector2/14 -> velocityIntegralLimitRHFE/1  "<velocityIntegralLimit>"
  Bus Selector2/13 -> velocityKdRHFE/1  "<velocityKd>"
  Bus Selector2/12 -> velocityKiRHFE/1  "<velocityKi>"
  Bus Selector2/11 -> velocityKpRHFE/1  "<velocityKp>"
  Bus Selector2/10 -> positionIntegralLimitRHFE/1  "<positionIntegralLimit>"
  Bus Selector2/9 -> positionKdRHFE/1  "<positionKd>"
  Bus Selector2/8 -> "positionKiRHFE "/1  "<positionKi>"
  Bus Selector2/7 -> positionKpRHFE/1  "<positionKp>"
  Bus Selector2/6 -> maxTorqueRHFE/1  "<maxTorque>"
  Bus Selector2/5 -> maxSpeedRHFE/1  "<maxSpeed>"
  Bus Selector2/4 -> maxPosLimitRHFE/1  "<maxPosLimit>"
  Bus Selector2/3 -> minPosLimitRHFE/1  "<minPosLimit>"
  Bus Selector2/2 -> polePairsRHFE/1  "<polePairs>"
  Bus Selector2/1 -> angleOffsetRHFE/1  "<angleOffset>"
  DemuxJointInfo2/3 -> Bus Selector2/1
  softStopThresholdLKFE/1 -> Out30/1
  velocityIntegralLimitLKFE/1 -> Out29/1
  velocityKdLKFE/1 -> Out28/1
  velocityKiLKFE/1 -> Out27/1
  velocityKpLKFE/1 -> Out26/1
  positionIntegralLimitLKFE/1 -> Out25/1
  positionKdLKFE/1 -> Out24/1
  positionKiLKFE/1 -> Out23/1
  positionKpLKFE/1 -> Out22/1
  maxTorqueLKFE/1 -> Out21/1
  maxSpeedLKFE/1 -> Out20/1
  maxPosLimitLFKE/1 -> Out19/1
  minPosLimitLKFE/1 -> Out18/1
  polePairsLKFE/1 -> Out17/1
  angleOffsetLKFE/1 -> Out16/1
  Bus Selector1/15 -> softStopThresholdLKFE/1  "<softStopThreshold>"
  Bus Selector1/14 -> velocityIntegralLimitLKFE/1  "<velocityIntegralLimit>"
  Bus Selector1/13 -> velocityKdLKFE/1  "<velocityKd>"
  Bus Selector1/12 -> velocityKiLKFE/1  "<velocityKi>"
  Bus Selector1/11 -> velocityKpLKFE/1  "<velocityKp>"
  Bus Selector1/10 -> positionIntegralLimitLKFE/1  "<positionIntegralLimit>"
  Bus Selector1/9 -> positionKdLKFE/1  "<positionKd>"
  Bus Selector1/8 -> positionKiLKFE/1  "<positionKi>"
  Bus Selector1/7 -> positionKpLKFE/1  "<positionKp>"
  Bus Selector1/6 -> maxTorqueLKFE/1  "<maxTorque>"
  Bus Selector1/5 -> maxSpeedLKFE/1  "<maxSpeed>"
  Bus Selector1/4 -> maxPosLimitLFKE/1  "<maxPosLimit>"
  Bus Selector1/3 -> minPosLimitLKFE/1  "<minPosLimit>"
  Bus Selector1/2 -> polePairsLKFE/1  "<polePairs>"
  Bus Selector1/1 -> angleOffsetLKFE/1  "<angleOffset>"
  DemuxJointInfo2/2 -> Bus Selector1/1
  softStopThresholdLHFE/1 -> Out15/1
  velocityIntegralLimitLHFE/1 -> Out14/1
  velocityKdLHFE/1 -> Out13/1
  velocityKiLHFE/1 -> Out12/1
  velocityKpLHFE/1 -> Out11/1
  positionIntegralLimitLHFE/1 -> Out10/1
  positionKdLHFE/1 -> Out9/1
  positionKiLHFE/1 -> Out8/1
  positionKpLHFE/1 -> Out7/1
  maxTorqueLHFE/1 -> Out6/1
  maxSpeedLHFE/1 -> Out5/1
  maxPosLimitLHFE/1 -> Out4/1
  minPosLimitLHFE/1 -> Out3/1
  polePairsLHFE/1 -> Out2/1
  angleOffsetLHFE/1 -> Out1/1
  Bus Selector/15 -> softStopThresholdLHFE/1  "<softStopThreshold>"
  Bus Selector/14 -> velocityIntegralLimitLHFE/1  "<velocityIntegralLimit>"
  Bus Selector/13 -> velocityKdLHFE/1  "<velocityKd>"
  Bus Selector/12 -> velocityKiLHFE/1  "<velocityKi>"
  Bus Selector/11 -> velocityKpLHFE/1  "<velocityKp>"
  Bus Selector/10 -> positionIntegralLimitLHFE/1  "<positionIntegralLimit>"
  Bus Selector/9 -> positionKdLHFE/1  "<positionKd>"
  Bus Selector/8 -> positionKiLHFE/1  "<positionKi>"
  Bus Selector/7 -> positionKpLHFE/1  "<positionKp>"
  Bus Selector/6 -> maxTorqueLHFE/1  "<maxTorque>"
  Bus Selector/5 -> maxSpeedLHFE/1  "<maxSpeed>"
  Bus Selector/4 -> maxPosLimitLHFE/1  "<maxPosLimit>"
  Bus Selector/3 -> minPosLimitLHFE/1  "<minPosLimit>"
  Bus Selector/2 -> polePairsLHFE/1  "<polePairs>"
  Bus Selector/1 -> angleOffsetLHFE/1  "<angleOffset>"
  DemuxJointInfo2/1 -> Bus Selector/1
  In1/1 -> DemuxJointInfo2/1

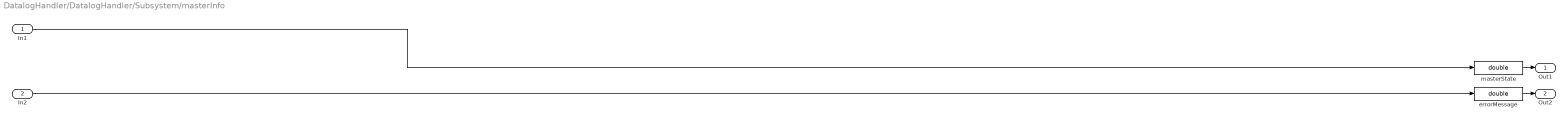
== system DatalogHandler/DatalogHandler/Subsystem/masterInfo ==
  In1 : Inport
  In2 : Inport  Port=2
  errorMessage : DataTypeConversion  OutDataTypeStr=double  RndMeth=Nearest
  masterState : DataTypeConversion  OutDataTypeStr=double  RndMeth=Nearest
  Out1 : Outport
  Out2 : Outport  Port=2
  wires:
  In1/1 -> masterState/1
  errorMessage/1 -> Out2/1
  masterState/1 -> Out1/1
  In2/1 -> errorMessage/1

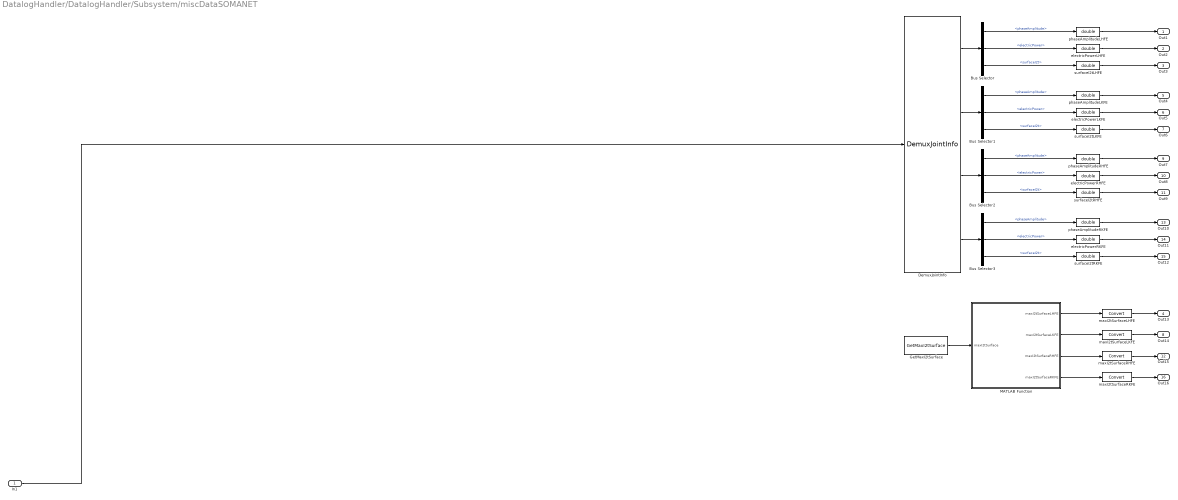
== system DatalogHandler/DatalogHandler/Subsystem/miscDataSOMANET ==
  In1 : Inport
  Bus Selector{,1..3} (4 alike) : BusSelector  OutputSignals=phaseAmplitude,electricPower,surfaceI2t
  DemuxJointInfo : VariousLibrary/DemuxJointInfo
  GetMaxI2tSurface : VariousLibrary/GetMaxI2tSurface
  MATLAB Function : MATLAB Function  TreatAsAtomicUnit=on
  electricPowerLHFE : DataTypeConversion  OutDataTypeStr=double  RndMeth=Nearest
  electricPowerLKFE : DataTypeConversion  OutDataTypeStr=double  RndMeth=Nearest
  electricPowerRHFE : DataTypeConversion  OutDataTypeStr=double  RndMeth=Nearest
  electricPowerRKFE : DataTypeConversion  OutDataTypeStr=double  RndMeth=Nearest
  maxI2tSurfaceLHFE : DataTypeConversion
  maxI2tSurfaceLKFE : DataTypeConversion
  maxI2tSurfaceRHFE : DataTypeConversion
  maxI2tSurfaceRKFE : DataTypeConversion
  phaseAmplitudeLHFE : DataTypeConversion  OutDataTypeStr=double  RndMeth=Nearest
  phaseAmplitudeLKFE : DataTypeConversion  OutDataTypeStr=double  RndMeth=Nearest
  phaseAmplitudeRHFE : DataTypeConversion  OutDataTypeStr=double  RndMeth=Nearest
  phaseAmplitudeRKFE : DataTypeConversion  OutDataTypeStr=double  RndMeth=Nearest
  surfaceI2tLHFE : DataTypeConversion  OutDataTypeStr=double  RndMeth=Nearest
  surfaceI2tLKFE : DataTypeConversion  OutDataTypeStr=double  RndMeth=Nearest
  surfaceI2tRHFE : DataTypeConversion  OutDataTypeStr=double  RndMeth=Nearest
  surfaceI2tRKFE : DataTypeConversion  OutDataTypeStr=double  RndMeth=Nearest
  Out1 : Outport
  Out2 : Outport  Port=2
  Out3 : Outport  Port=3
  Out13 : Outport  Port=4
  Out4 : Outport  Port=5
  Out5 : Outport  Port=6
  Out6 : Outport  Port=7
  Out14 : Outport  Port=8
  Out7 : Outport  Port=9
  Out8 : Outport  Port=10
  Out9 : Outport  Port=11
  Out15 : Outport  Port=12
  Out10 : Outport  Port=13
  Out11 : Outport  Port=14
  Out12 : Outport  Port=15
  Out16 : Outport  Port=16
  wires:
  maxI2tSurfaceLHFE/1 -> Out13/1
  maxI2tSurfaceLKFE/1 -> Out14/1
  maxI2tSurfaceRHFE/1 -> Out15/1
  maxI2tSurfaceRKFE/1 -> Out16/1
  MATLAB Function/4(maxI2tSurfaceRKFE) -> maxI2tSurfaceRKFE/1
  MATLAB Function/3(maxI2tSurfaceRHFE) -> maxI2tSurfaceRHFE/1
  MATLAB Function/2(maxI2tSurfaceLKFE) -> maxI2tSurfaceLKFE/1
  MATLAB Function/1(maxI2tSurfaceLHFE) -> maxI2tSurfaceLHFE/1
  GetMaxI2tSurface/1 -> MATLAB Function/1(maxI2tSurface)
  electricPowerLHFE/1 -> Out2/1
  surfaceI2tLHFE/1 -> Out3/1
  phaseAmplitudeLKFE/1 -> Out4/1
  electricPowerLKFE/1 -> Out5/1
  surfaceI2tLKFE/1 -> Out6/1
  phaseAmplitudeRHFE/1 -> Out7/1
  electricPowerRHFE/1 -> Out8/1
  surfaceI2tRHFE/1 -> Out9/1
  phaseAmplitudeRKFE/1 -> Out10/1
  electricPowerRKFE/1 -> Out11/1
  surfaceI2tRKFE/1 -> Out12/1
  phaseAmplitudeLHFE/1 -> Out1/1
  Bus Selector3/3 -> surfaceI2tRKFE/1  "<surfaceI2t>"
  Bus Selector3/2 -> electricPowerRKFE/1  "<electricPower>"
  Bus Selector3/1 -> phaseAmplitudeRKFE/1  "<phaseAmplitude>"
  Bus Selector2/3 -> surfaceI2tRHFE/1  "<surfaceI2t>"
  Bus Selector2/1 -> phaseAmplitudeRHFE/1  "<phaseAmplitude>"
  Bus Selector2/2 -> electricPowerRHFE/1  "<electricPower>"
  Bus Selector1/3 -> surfaceI2tLKFE/1  "<surfaceI2t>"
  Bus Selector1/2 -> electricPowerLKFE/1  "<electricPower>"
  Bus Selector1/1 -> phaseAmplitudeLKFE/1  "<phaseAmplitude>"
  Bus Selector/3 -> surfaceI2tLHFE/1  "<surfaceI2t>"
  Bus Selector/2 -> electricPowerLHFE/1  "<electricPower>"
  Bus Selector/1 -> phaseAmplitudeLHFE/1  "<phaseAmplitude>"
  DemuxJointInfo/4 -> Bus Selector3/1
  DemuxJointInfo/3 -> Bus Selector2/1
  DemuxJointInfo/2 -> Bus Selector1/1
  DemuxJointInfo/1 -> Bus Selector/1
  In1/1 -> DemuxJointInfo/1

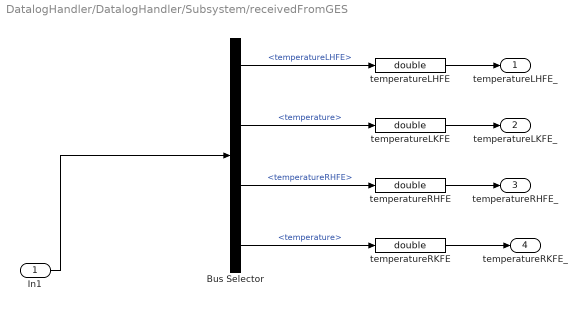
== system DatalogHandler/DatalogHandler/Subsystem/receivedFromGES ==
  In1 : Inport
  Bus Selector : BusSelector  OutputSignals=receivedFromGESBack.temperatureLHFE,receivedFromGESLKFE.temperature,receivedFromGESBack.temperatureRHFE,receivedFromGESRKFE.temperature
  temperatureLHFE : DataTypeConversion  OutDataTypeStr=double  RndMeth=Nearest
  temperatureLKFE : DataTypeConversion  OutDataTypeStr=double  RndMeth=Nearest
  temperatureRHFE : DataTypeConversion  OutDataTypeStr=double  RndMeth=Nearest
  temperatureRKFE : DataTypeConversion  OutDataTypeStr=double  RndMeth=Nearest
  temperatureLHFE_ : Outport
  temperatureLKFE_ : Outport  Port=2
  temperatureRHFE_ : Outport  Port=3
  temperatureRKFE_ : Outport  Port=4
  wires:
  temperatureLHFE/1 -> temperatureLHFE_/1
  temperatureRHFE/1 -> temperatureRHFE_/1
  temperatureLKFE/1 -> temperatureLKFE_/1
  temperatureRKFE/1 -> temperatureRKFE_/1
  In1/1 -> Bus Selector/1
  Bus Selector/1 -> temperatureLHFE/1  "<temperatureLHFE>"
  Bus Selector/3 -> temperatureRHFE/1  "<temperatureRHFE>"
  Bus Selector/2 -> temperatureLKFE/1  "<temperature>"
  Bus Selector/4 -> temperatureRKFE/1  "<temperature>"

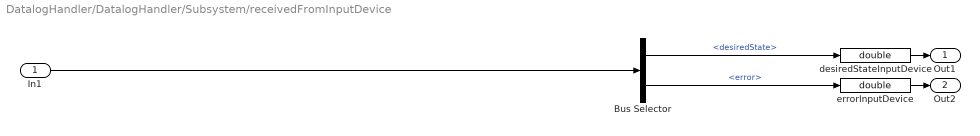
== system DatalogHandler/DatalogHandler/Subsystem/receivedFromInputDevice ==
  In1 : Inport
  Bus Selector : BusSelector  OutputSignals=desiredState,error
  desiredStateInputDevice : DataTypeConversion  OutDataTypeStr=double  RndMeth=Nearest
  errorInputDevice : DataTypeConversion  OutDataTypeStr=double  RndMeth=Nearest
  Out1 : Outport
  Out2 : Outport  Port=2
  wires:
  In1/1 -> Bus Selector/1
  Bus Selector/2 -> errorInputDevice/1  "<error>"
  Bus Selector/1 -> desiredStateInputDevice/1  "<desiredState>"
  desiredStateInputDevice/1 -> Out1/1
  errorInputDevice/1 -> Out2/1

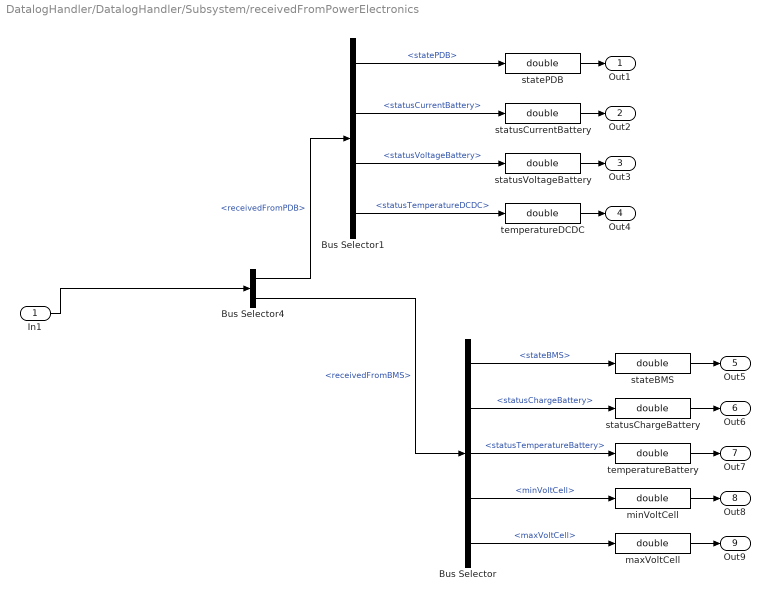
== system DatalogHandler/DatalogHandler/Subsystem/receivedFromPowerElectronics ==
  In1 : Inport
  Bus Selector : BusSelector  OutputSignals=stateBMS,statusChargeBattery,statusTemperatureBattery,minVoltCell,maxVoltCell
  Bus Selector1 : BusSelector  OutputSignals=statePDB,statusCurrentBattery,statusVoltageBattery,statusTemperatureDCDC
  Bus Selector4 : BusSelector  OutputSignals=receivedFromPDB,receivedFromBMS
  maxVoltCell : DataTypeConversion  OutDataTypeStr=double  RndMeth=Nearest
  minVoltCell : DataTypeConversion  OutDataTypeStr=double  RndMeth=Nearest
  stateBMS : DataTypeConversion  OutDataTypeStr=double  RndMeth=Nearest
  statePDB : DataTypeConversion  OutDataTypeStr=double  RndMeth=Nearest
  statusChargeBattery : DataTypeConversion  OutDataTypeStr=double  RndMeth=Nearest
  statusCurrentBattery : DataTypeConversion  OutDataTypeStr=double  RndMeth=Nearest
  statusVoltageBattery : DataTypeConversion  OutDataTypeStr=double  RndMeth=Nearest
  temperatureBattery : DataTypeConversion  OutDataTypeStr=double  RndMeth=Nearest
  temperatureDCDC : DataTypeConversion  OutDataTypeStr=double  RndMeth=Nearest
  Out1 : Outport
  Out2 : Outport  Port=2
  Out3 : Outport  Port=3
  Out4 : Outport  Port=4
  Out5 : Outport  Port=5
  Out6 : Outport  Port=6
  Out7 : Outport  Port=7
  Out8 : Outport  Port=8
  Out9 : Outport  Port=9
  wires:
  maxVoltCell/1 -> Out9/1
  minVoltCell/1 -> Out8/1
  temperatureBattery/1 -> Out7/1
  statusChargeBattery/1 -> Out6/1
  stateBMS/1 -> Out5/1
  temperatureDCDC/1 -> Out4/1
  statusVoltageBattery/1 -> Out3/1
  statusCurrentBattery/1 -> Out2/1
  statePDB/1 -> Out1/1
  Bus Selector/5 -> maxVoltCell/1  "<maxVoltCell>"
  Bus Selector/4 -> minVoltCell/1  "<minVoltCell>"
  Bus Selector/3 -> temperatureBattery/1  "<statusTemperatureBattery>"
  Bus Selector/2 -> statusChargeBattery/1  "<statusChargeBattery>"
  Bus Selector/1 -> stateBMS/1  "<stateBMS>"
  Bus Selector1/4 -> temperatureDCDC/1  "<statusTemperatureDCDC>"
  Bus Selector1/3 -> statusVoltageBattery/1  "<statusVoltageBattery>"
  Bus Selector1/2 -> statusCurrentBattery/1  "<statusCurrentBattery>"
  Bus Selector1/1 -> statePDB/1  "<statePDB>"
  Bus Selector4/2 -> Bus Selector/1  "<receivedFromBMS>"
  In1/1 -> Bus Selector4/1
  Bus Selector4/1 -> Bus Selector1/1  "<receivedFromPDB>"
